simulink model "multiTether_th"  (R2018b)
settings: Solver=VariableStepAuto  StartTime=0.0  StopTime=10.0  RelTol=1e-3
undefined symbols (not defined in the file or in its folder): node_locations
settings Model: Creator=mcobb  LastModifiedBy=mcobb

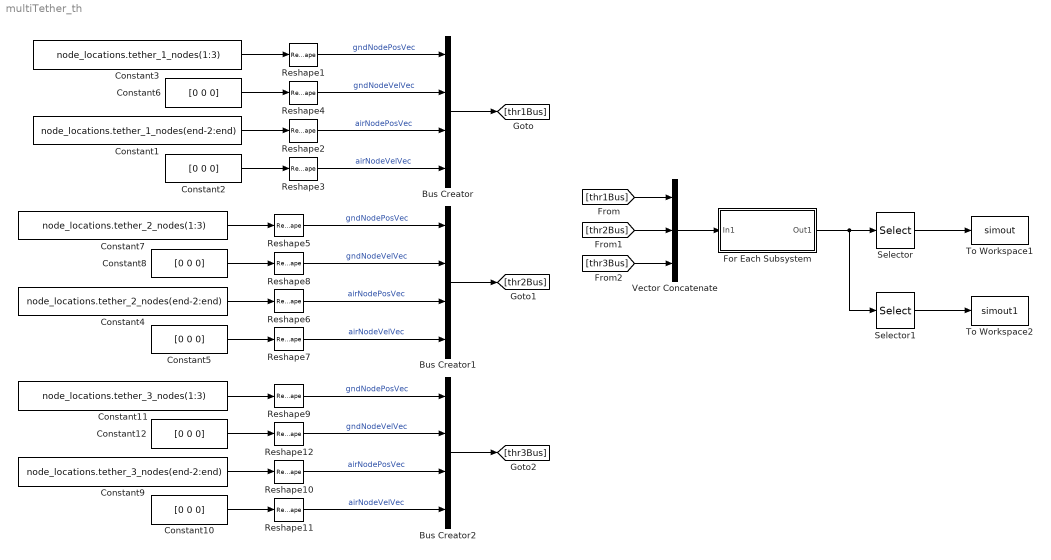
== system multiTether_th ==
  Bus Creator : BusCreator  Inputs=4  OutDataTypeStr=Bus: tetherInputBus  NonVirtualBus=on
  Bus Creator1 : BusCreator  Inputs=4  OutDataTypeStr=Bus: tetherInputBus  NonVirtualBus=on
  Bus Creator2 : BusCreator  Inputs=4  OutDataTypeStr=Bus: tetherInputBus  NonVirtualBus=on
  Constant1 : Constant  Value=node_locations.tether_1_nodes(end-2:end)
  Constant{2,5..6,8,10,12} (6 alike) : Constant  Value=[0 0 0]
  Constant11 : Constant  Value=node_locations.tether_3_nodes(1:3)
  Constant3 : Constant  Value=node_locations.tether_1_nodes(1:3)
  Constant4 : Constant  Value=node_locations.tether_2_nodes(end-2:end)
  Constant7 : Constant  Value=node_locations.tether_2_nodes(1:3)
  Constant9 : Constant  Value=node_locations.tether_3_nodes(end-2:end)
  For Each Subsystem : Subsystem  TreatAsAtomicUnit=on
  Reshape{1..12} (12 alike) : Reshape  OutputDimensionality=Column vector (2-D)
  Selector : Selector  InputPortWidth=3  IndexOptions=Index vector (dialog)  Indices=1  OutputSizes=1
  Selector1 : Selector  InputPortWidth=3  IndexOptions=Index vector (dialog)  Indices=2  OutputSizes=1
  To Workspace1 : ToWorkspace  VariableName=simout  SaveFormat=Timeseries  SampleTime=-1
  To Workspace2 : ToWorkspace  VariableName=simout1  SaveFormat=Timeseries  SampleTime=-1
  Vector Concatenate : Concatenate  NumInputs=3
  wires:
  Constant3/1 -> Reshape1/1
  Reshape1/1 -> Bus Creator/1  "gndNodePosVec"
  Vector Concatenate/1 -> For Each Subsystem/1(In1)
  For Each Subsystem/1(Out1) -> Selector1/1, Selector/1
  Constant6/1 -> Reshape4/1
  Bus Creator/1 -> [thr1Bus]
  [thr1Bus] -> Vector Concatenate/1
  [thr2Bus] -> Vector Concatenate/2
  [thr3Bus] -> Vector Concatenate/3
  Selector/1 -> To Workspace1/1
  Reshape4/1 -> Bus Creator/2  "gndNodeVelVec"
  Reshape2/1 -> Bus Creator/3  "airNodePosVec"
  Constant1/1 -> Reshape2/1
  Constant2/1 -> Reshape3/1
  Reshape3/1 -> Bus Creator/4  "airNodeVelVec"
  Reshape7/1 -> Bus Creator1/4  "airNodeVelVec"
  Constant5/1 -> Reshape7/1
  Constant4/1 -> Reshape6/1
  Reshape6/1 -> Bus Creator1/3  "airNodePosVec"
  Reshape8/1 -> Bus Creator1/2  "gndNodeVelVec"
  Bus Creator1/1 -> [thr2Bus]
  Constant8/1 -> Reshape8/1
  Reshape5/1 -> Bus Creator1/1  "gndNodePosVec"
  Constant7/1 -> Reshape5/1
  Constant11/1 -> Reshape9/1
  Reshape9/1 -> Bus Creator2/1  "gndNodePosVec"
  Constant12/1 -> Reshape12/1
  Bus Creator2/1 -> [thr3Bus]
  Reshape12/1 -> Bus Creator2/2  "gndNodeVelVec"
  Reshape10/1 -> Bus Creator2/3  "airNodePosVec"
  Constant9/1 -> Reshape10/1
  Constant10/1 -> Reshape11/1
  Reshape11/1 -> Bus Creator2/4  "airNodeVelVec"
  Selector1/1 -> To Workspace2/1

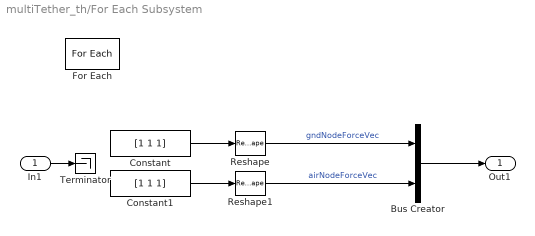
== system multiTether_th/For Each Subsystem ==
  In1 : Inport  Partition=on  PartitionDimension=1  PartitionWidth=1  PartitionOffset=0
  Bus Creator : BusCreator  Inputs=2  OutDataTypeStr=Bus: tetherOutputBus  NonVirtualBus=on
  Constant : Constant  Value=[1 1 1]
  Constant1 : Constant  Value=[1 1 1]
  For Each : ForEach  DisableCoverage=on  IndexMode=One-based
  Reshape : Reshape  OutputDimensionality=Column vector (2-D)
  Reshape1 : Reshape  OutputDimensionality=Column vector (2-D)
  Terminator : Terminator
  Out1 : Outport  ConcatenationDimension=1
  wires:
  In1/1 -> Terminator/1
  Bus Creator/1 -> Out1/1
  Constant/1 -> Reshape/1
  Reshape/1 -> Bus Creator/1  "gndNodeForceVec"
  Constant1/1 -> Reshape1/1
  Reshape1/1 -> Bus Creator/2  "airNodeForceVec"
